simulink model "motor"  (Simulink 3.00)
libraries: mathlib x8, genlib x2, arclib x1

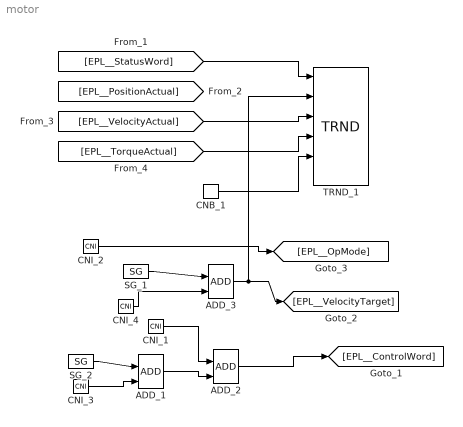
== system motor ==
  ADD_1 : mathlib/ADD
  ADD_2 : mathlib/ADD
  ADD_3 : mathlib/ADD
  CNB_1 : mathlib/CNB  YCN=on
  CNI_1 : mathlib/CNI  icn=15
  CNI_2 : mathlib/CNI  icn=3
  CNI_3 : mathlib/CNI  icn=64
  CNI_4 : mathlib/CNI  icn=0
  SG_1 : genlib/SG  isig=1: SINE  amp=0  freq=0.05  phase=0  ifrunit=1: Hz  iphunit=1: degree
  SG_2 : genlib/SG  isig=2: SQUARE  amp=64  freq=0.1  phase=0  ifrunit=1: Hz  iphunit=1: degree
  TRND_1 : arclib/TRND  n=4  l=1000  btype=8: Double  ptype1=1: Store  ptype2=1: Store  ptype3=1: Store  ptype4=1: Store  pfac=1  afac=0  arc=0  id=1  Title=Trend Title
  wires:
  ADD_1/1 -> ADD_2/2
  ADD_2/1 -> [EPL__ControlWord]
  ADD_3/1 -> [EPL__VelocityTarget], TRND_1/2
  CNB_1/1 -> TRND_1/5
  CNI_1/1 -> ADD_2/1
  CNI_2/1 -> [EPL__OpMode]
  CNI_3/1 -> ADD_1/2
  CNI_4/1 -> ADD_3/2
  [EPL__StatusWord] -> TRND_1/1
  [EPL__VelocityActual] -> TRND_1/3
  [EPL__TorqueActual] -> TRND_1/4
  SG_1/1 -> ADD_3/1
  SG_2/1 -> ADD_1/1
